simulink model "SensorModel"  (R2026a)
settings: Solver=FixedStepAuto  StartTime=0  StopTime=1000  FixedStep=0.1
model workspace (MAT data in the model file):
  SL_ROS_VariableLengthArrays_MaxSizes.CommonInfo.ArrayTruncateAction = 'EmitWarning'
  SL_ROS_VariableLengthArrays_MaxSizes.MsgTypeMap = containers.Map
  SL_ROS_VariableLengthArrays_MaxSizes.MsgTypeMap.serialization.keys = {'sensor_msgs/PointCloud2'}
  SL_ROS_VariableLengthArrays_MaxSizes.MsgTypeMap.serialization.values{1}(1).PropertyName = 'data'
  SL_ROS_VariableLengthArrays_MaxSizes.MsgTypeMap.serialization.values{1}(1).DataType = 'uint8'
  SL_ROS_VariableLengthArrays_MaxSizes.MsgTypeMap.serialization.values{1}(1).MaxLength = 4915200
  SL_ROS_VariableLengthArrays_MaxSizes.MsgTypeMap.serialization.values{1}(2).PropertyName = 'fields'
  SL_ROS_VariableLengthArrays_MaxSizes.MsgTypeMap.serialization.values{1}(2).DataType = 'sensor_msgs/PointField'
  SL_ROS_VariableLengthArrays_MaxSizes.MsgTypeMap.serialization.values{1}(2).MaxLength = 16
  SL_ROS_VariableLengthArrays_MaxSizes.MsgTypeMap.serialization.uniformity = 0
  SL_ROS_VariableLengthArrays_MaxSizes.MsgTypeMap.serialization.keyType = 'char'
  SL_ROS_VariableLengthArrays_MaxSizes.MsgTypeMap.serialization.valueType = 'any'
undefined symbols (not defined in the file): Defined, Ego, Lane, matlabshared, Sim3dSensor, simStepSize, User
libraries: roadrunnerscenario x6, drivingscenarioandsensors x2, ros2lib x2, sensoridealgroundtruthlib x1, sim3dcameralib x1, sim3dlib x1, sim3dautolib x1
settings Model: Creator=The MathWorks, Inc.  LastModifiedBy=akshran
settings DataIOCC: MaxDataPoints=100  SaveFormat=StructureWithTime  DatasetSignalFormat=timetable
settings DebuggingCC: SubsystemReferenceDiagnosticForUnitTest=warning
settings RTWCC: SystemTargetFile=ert.tlc  HardwareBoard=Robot Operating System 2 (ROS 2)  TLCOptions="-aInlineSetEventsForThisBaseRateFcn=TLC_FALSE -aSuppressMultiTaskScheduler=TLC_FALSE  -aRateBasedStepFcn=0"  Toolchain=Colcon Tools  TargetLang=C++  Description=Embedded Coder
settings ERTTargetCC: ExtModeTransport=2.0  ExtModeAutomaticAllocSize=off  RootIOFormat=Structure reference  CodeInterfacePackaging=C++ class

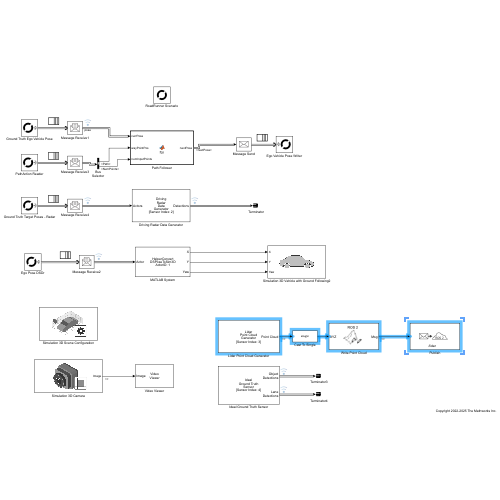
[thumbnail: Simulink's stored preview of the top-level diagram]
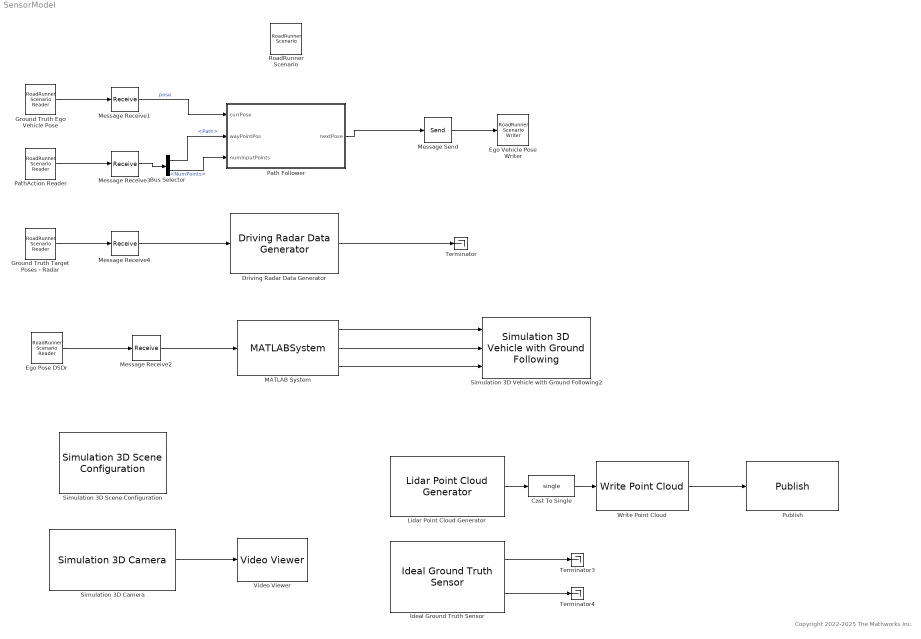
== system SensorModel ==
  note: Copyright 2022-2025 The Mathworks Inc.
  Bus Selector : BusSelector  OutputSignals=PathTarget.Path,PathTarget.NumPoints
  Cast To Single : DataTypeConversion  OutDataTypeStr=single  SaturateOnIntegerOverflow=off  RndMeth=Floor
  Driving Radar Data Generator : drivingscenarioandsensors/Driving Radar Data Generator  SensorIndex=2  UpdateRate=1/simStepSize  MountingLocation=[1.8, 0, 0.2 ]  MountingAngles=[0 0 0]  HasElevation=off  HasRangeRate=on  HasNoise=on  HasFalseAlarms=on  HasOcclusion=on  MaxNumReportsSource=Property  MaxNumReports=50  TargetReportFormat=Detections  DetectionCoordinates=Body  TrackCoordinates=Body  BusNameSource=Auto  BusName=BusDrivingRadarDataGenerator  SimulateUsing=Interpreted execution  AzimuthResolution=1  ElevationResolution=5  RangeResolution=2.5  RangeRateResolution=0.5  AzimuthBiasFraction=0.1  ElevationBiasFraction=0.1  RangeBiasFraction=0.05  RangeRateBiasFraction=0.05  FieldOfView=[ 80, 5 ]  RangeLimits=[ 0, 150 ]  RangeRateLimits=[ -100, 100 ]  DetectionProbability=0.9  FalseAlarmRate=1e-06  ReferenceRange=100  ReferenceRCS=0  CenterFrequency=77e9  FilterInitializationFcn=initcvekf  ConfirmationThreshold=[2 3]  DeletionThreshold=[5 5]  InitialSeedSource=Repeatable  InitialSeed=0  UsedSeed=matlabshared.tracking.internal.SimulinkUtilities.seedManager(gcb)  ProfilesSource=From Scenario Reader block  ProfilesParameters=driving.internal.ActorProfilesRadarParameters  ProfilesExpression=struct('ClassID',0,'Length',4.7,'Width',1.8,'Height',1.4,'OriginOffset',[-1.35 0 0],'RCSPattern',[10 10;10 10],'RCSAzimuthAngles',[-180 180],'RCSElevationAngles',[-90 90])
  Ego Pose DSDr : roadrunnerscenario/RoadRunner Scenario Reader  TopicCategory=Actor  ActorCategory=All Types  ActionType=Path Following  EventType=User-Defined  TopicType=Actor Pose (Driving Scenario compatible)  VehicleType=Vehicle Specifications  TrafficSignalType=Traffic Signal Specifications  TrafficSignalControllerType=Traffic Signal Controller Specifications  UserDefinedAction=Action1  UserDefinedEvent=Event1  Filter=Self  AdditionalRelationship=None  SensorTopic=Target Poses  LaneBoundaryOutputTopic=Ego-Lane  SensorID=1  SampleTime=0.1
  Ego Vehicle Pose Writer : roadrunnerscenario/RoadRunner Scenario Writer  TopicCategory=Actor  ActorCategory=All Types  EventType=Action Complete  UserDefinedEvent=Event1  VehicleType=Vehicle Pose  TopicType=Actor Pose
  Ground Truth Ego Vehicle Pose : roadrunnerscenario/RoadRunner Scenario Reader  TopicCategory=Actor  ActorCategory=All Types  ActionType=Path Following  EventType=User-Defined  TopicType=Actor Pose  VehicleType=Vehicle Pose  TrafficSignalType=Traffic Signal Specifications  TrafficSignalControllerType=Traffic Signal Controller Specifications  UserDefinedAction=Action1  UserDefinedEvent=Event1  Filter=Self  AdditionalRelationship=None  SensorTopic=Target Poses  LaneBoundaryOutputTopic=Ego-Lane  SensorID=1  SampleTime=0.1
  Ground Truth Target Poses - Radar : roadrunnerscenario/RoadRunner Scenario Reader  TopicCategory=Sensor  ActorCategory=All Types  ActionType=Path Following  EventType=User-Defined  TopicType=Actor Specifications  VehicleType=Vehicle Specifications  TrafficSignalType=Traffic Signal Specifications  TrafficSignalControllerType=Traffic Signal Controller Specifications  UserDefinedAction=Action1  UserDefinedEvent=Event1  Filter=Self  AdditionalRelationship=None  SensorTopic=Target Poses  LaneBoundaryOutputTopic=Ego-Lane  SensorID=2  SampleTime=0.1
  Ideal Ground Truth Sensor : sensoridealgroundtruthlib/Ideal Ground Truth Sensor  SensorIndex=4  DetectorOutput=Objects and Lanes  UpdateInterval=simStepSize  SensorLocation=[ 1.9, 0, 0.2 ]  Yaw=0  Pitch=0  Roll=0  FieldOfView=[ 120, 30 ]  MaxRange=50  DetectionCoordinates=Host Coordinates  PointOnTargetReported=Origin Point  TargetOutputFormat=Object Detections  MaxNumObjectDetections=300  LaneBoundariesReported=All Lanes  MaxNumLaneDetections=300  BusNameSource=Auto  BusName=BusSSFGroundTruthObjects  BusName2Source=Auto  BusName2=BusSSFGroundTruthLaneBoundaries  SimulateUsing=Interpreted execution
  Lidar Point Cloud Generator : drivingscenarioandsensors/Lidar Point Cloud Generator  SensorIndex=3  UpdateInterval=simStepSize  SensorLocation=[1.5 0]  Height=1.6  Yaw=0  Pitch=0  Roll=0  DetectionCoordinates=Ego Cartesian  HasEgoVehicle=on  EgoVehicleActorID=1  HasRoadsInputPort=on  ActorProfilesSource=From Scenario Reader block  ActorProfilesVariableName=actor_profiles  MaxRange=120  RangeAccuracy=0.002  AzimuthResolution=0.16  ElevationResolution=1.25  AzimuthLimits=[ -180, 180 ]  ElevationLimits=[ -20, 20 ]  HasNoise=on
  MATLAB System : MATLABSystem  System=HelperConvertDSPoseToSim3D  ActorProfiles=struct( 'ActorID', 1, 'ClassID', 1, 'Length', 4.7, 'Width', 1.8, 'Height', 1.4, 'OriginOffset', [ 0, 0, 0 ], 'FrontOverhang', 0, 'RearOverhang', 0, 'Wheelbase', 0, 'Color', [ 0, 0, 0 ] )  ActorIDToConvert=1  SimulateUsing=Code generation
      mask Type: HelperConvertDSPoseToSim3D
  Message Receive{1..4} (4 alike) : Receive  InputPortMessageModes=m  UseInternalQueue=off  SampleTime=simStepSize
  Message Send : Send  OutputPortMessageModes=m
  Path Follower : MATLAB Function  TreatAsAtomicUnit=on
  PathAction Reader : roadrunnerscenario/RoadRunner Scenario Reader  TopicCategory=Action  ActorCategory=All Types  ActionType=Path Following  EventType=User-Defined  TopicType=Actor Specifications  VehicleType=Vehicle Specifications  TrafficSignalType=Traffic Signal Specifications  TrafficSignalControllerType=Traffic Signal Controller Specifications  UserDefinedAction=Action1  UserDefinedEvent=Event1  Filter=Self  AdditionalRelationship=None  SensorTopic=Target Poses  LaneBoundaryOutputTopic=Ego-Lane  SensorID=1  SampleTime=0.1
  Publish : ros2lib/Publish  topicSource=Specify your own  topic=/lidar  messageType=sensor_msgs/PointCloud2  QOSHistory=Keep last  QOSDepth=10  QOSReliability=Reliable  QOSDurability=Volatile  QOSDeadline=Inf  QOSLifespan=Inf  QOSLiveliness=Automatic  QOSLeaseDuration=Inf  QOSAvoidROSNamespaceConventions=off
  RoadRunner Scenario : roadrunnerscenario/RoadRunner Scenario  ScenarioFileName=C:\Users\akshran\OneDrive - MathWorks\Documents\EIC_RR1\EIC_FW\Scenarios\EIC  ActorIDLinkedToModel=1  SampleTime=0.1  OpenRoadRunnerAtSimulationStart=on  EnableSimulationLoggingInRoadRunner=on  UserDefinedActions={}  UserDefinedEvents={}  PathPoints=500
  Simulation 3D Camera : sim3dcameralib/Simulation 3D Camera  Priority=1  sensorTag=Sim3dSensor�  sensorId=1  sensorName=Sim3dSensor�  vehTagList={'Custom ...';'Scene Origin';'SimulinkVehicle1'}  vehTag=SimulinkVehicle1  CoordinateSystem=ISO8855  mountLoc=Roof center  offsetFlag=off  tmountOffset=[0, 0, 0]  extTmount=off  rmountOffset=[0, 0, 0]  extRmount=off  FocalLength=[1109, 1109]  OpticalCenter=[640, 360]  ImageSize=[720, 1280]  RadialDistortion=[0, 0]  TangentialDistortion=[0, 0]  SensorSkew=0  VisualizeFieldOfView=off  FieldOfViewRange=61  DepthOutportEnabled=off  SemanticOutportEnabled=off  TransformOutportEnabled=off  SampleTime=-1  mountPoint=[-0.45 0 1.68]  mountOrientation=[0 0 0]  aMode=3  ID=1
      settings: LibrarySourceBlock=drivingsim3d/Simulation 3D Camera
  Simulation 3D Scene Configuration : sim3dlib/Simulation 3D Scene Configuration  Priority=0  ProjectFormat=RoadRunner  SceneDesc=Straight road  ProjectName=C:\Program Files\MATLAB\R2026a\toolbox\shared\sim3d_projects\automotive_project_windows\UE\WindowsNoEditor\VehicleSimulation.exe  ScenePath=/Game/Maps/HwStrght  RoadRunnerProjectPath=C:\Users\akshran\OneDrive - MathWorks\Documents\EIC_RR1\EIC_FW\Exports\EIC.fbx  EnableOpenDRIVE=off  vehTagList={'Custom';'Scene Origin';'SimulinkVehicle1'}  vehTag=SimulinkVehicle1  AttachedCameraRelativeTranslation=[0 0 0]  FreeCameraDefaultInitialTranslation=[-6, 0, 2]  AttachedCameraRelativeRotation=[0, -15, 0]  FreeCameraDefaultInitialRotation=[0, -15, 0]  ViewpointName=Custom  FreeCameraInitialTranslation=[0, 0, 0]  FreeCameraInitialRotation=[0, 0, 0]  OpVisEn=off  Ts=0.1  EnableWindow=on  EnableRemoteAccess=off  SimulationMode=CoSimulation  SimulateUsing=Interpreted execution  EnableAnimationRecording=off  OverrideDefaultRecording=off  AnimationRecordingFileName=sim3dAnimation.mat  AnimationRecordingInterval=[0 inf]  EnableWeather=off  SunAzimuth=90  SunAltitude=40.0  EnableGeospatialSun=off  Latitude=0  Longitude=0  Date=2023-01-01  Time=10:30:00  GeoTimeZone=-5.0  SunDaylightSaving=off  wind=1  clouds=10  EnableVolumetricClouds=off  CloudCoverage=0  CloudAltitude=6  fog=0  rain=0  RaindropsEffect=off  SnowDensity=0  EnableGeospatial=off  TilesetSource=Earth terrain  UseTrueOrigin=off  OriginHeight=200  OriginLatitude=40.744652  OriginLongitude=-73.988864  MapStyle=Aerial  AdditionalAssetIDs=[]  UseAdvancedSunSky=off  SolarTime=11  TimeZone=-5  Day=21  Month=9  Year=2022  UseDaylightSavingTime=on  DSTStartDay=10  DSTStartMonth=3  DSTEndDay=3  DSTEndMonth=11  DSTSwitchHour=2  sensorTag=MainCamera1  sensorId=1  sensorName=MainCamera1  mountLoc=Origin  offsetFlag=off  tmountOffset=[0, 0, 0]  rmountOffset=[0, 0, 0]  HorizontalResolution=1280  VerticalResolution=720  HorizontalFOV=60  mountPoint=[0 0 0]  mountOrientation=[0 0 0]  aMode=3  ID=1  GeoTrigger=Inactive  ViewNameList={'Custom'}  ViewTranslationList={'[0 0 0]'}  ViewRotationList={'[0 0 0]'}
      settings: LibrarySourceBlock=drivingsim3d/Simulation 3D Scene Configuration
  Simulation 3D Vehicle with Ground Following2 : sim3dautolib/Simulation 3D Vehicle with Ground Following  Priority=-1  PassVehMesh=Sedan  MeshPath=/MathWorksAutomotiveContent/Vehicles/Muscle/Meshes/SK_MuscleCar.SK_MuscleCar  TrackWidth=1.9  WheelBase=3  WheelRadius=0.35  VehColor=Silver  CoordinateSystem=ISO8855  InitialPos=[-7.539,-70.4747,0]  InitialRot=[0, 0, 0]  ActorName=SimulinkVehicle1  SampleTime=-1  ActorType=SimulinkVehicle  ID=1  aMode=3  ActorTag=SimulinkVehicle1  CoordinateScheme=0  VehLightsControl=off  HeadlightColor=[ 1, 1, 1 ]  HighBeamIntensity=100000  LowBeamIntensity=60000  HighBeamConeAngle=70  LowBeamConeAngle=70  LeftHeadlightOrientation=[ 0, 0 ]  RightHeadlightOrientation=[ 0, 0 ]  BrakelightIntensity=500  ReverselightIntensity=500  SignallightIntensity=500  SignallightPeriod=1  SignalPulseWidth=50  TransformOutportEnabled=off
      settings: LibrarySourceBlock=drivingsim3d/Simulation 3D Vehicle with Ground Following
  Terminator : Terminator
  Terminator3 : Terminator
  Terminator4 : Terminator
  Video Viewer : VideoViewer  FigPos=[431 551 418 304]
  Write Point Cloud : ros2lib/Write Point Cloud  messageType=sensor_msgs/PointCloud2  Encoding=none  HasRGB=false  HasAlpha=false  HasIntensityCheck=off  HasIntensity=false  FieldNamesStruct=struct('x', 'single', 'y', 'single', 'z', 'single')
  wires:
  Ground Truth Ego Vehicle Pose/1 -> Message Receive1/1
  Path Follower/1(nextPose) -> Message Send/1
  Message Receive1/1 -> Path Follower/1(currPose)  "pose"
  PathAction Reader/1 -> Message Receive3/1
  Message Receive3/1 -> Bus Selector/1
  Message Send/1 -> Ego Vehicle Pose Writer/1
  Bus Selector/1 -> Path Follower/2(wayPointPos)  "<Path>"
  Driving Radar Data Generator/1 -> Terminator/1
  Ground Truth Target Poses - Radar/1 -> Message Receive4/1
  Message Receive4/1 -> Driving Radar Data Generator/1
  Lidar Point Cloud Generator/1 -> Cast To Single/1
  Ideal Ground Truth Sensor/1 -> Terminator3/1
  Ideal Ground Truth Sensor/2 -> Terminator4/1
  Bus Selector/2 -> Path Follower/3(numInputPoints)  "<NumPoints>"
  Simulation 3D Camera/1 -> Video Viewer/1
  Write Point Cloud/1 -> Publish/1
  Cast To Single/1 -> Write Point Cloud/1
  Message Receive2/1 -> MATLAB System/1
  Ego Pose DSDr/1 -> Message Receive2/1
  MATLAB System/1 -> Simulation 3D Vehicle with Ground Following2/1
  MATLAB System/2 -> Simulation 3D Vehicle with Ground Following2/2
  MATLAB System/3 -> Simulation 3D Vehicle with Ground Following2/3

== matlab function SensorModel/Path Follower ==
  data: currPose input; wayPointPos input; numInputPoints input; nextPose output Bus: BusActorRuntime; simStepSize parameter
function nextPose    = fcn(currPose, wayPointPos, numInputPoints, simStepSize)

% Set constant ego vehicle speed
egoSpeed  = 18;

% Declare persistent variables for simulation and retain only non zero
% elements in the array of waypoints 
persistent wayPointIdx wayPointPosInterp headingAnglesInterp numWayPoints
wayPointPos = wayPointPos(1:numInputPoints,:);

% Extract poses for the entire path before simulation begins
if isempty(wayPointIdx)
    
    wayPointIdx = 2;

    % Pre-allocate arrays
    wayPointPosInterp = [];
    headingAnglesInterp = [];

    % Get heading angle
    startHeadingAngle = atan2d(-currPose.Pose(1,2),currPose.Pose(1,1));
  
     % Calculate distance from the each waypoint to the next waypoint
    delXY = diff(wayPointPos(:,[1 2]));
    absDistToNextPoints = sqrt(delXY(:,1).^2 + delXY(:,2).^2);

    % Calculate time of arrival at the next wayPoint based on the
    % set constant speed. Alternatively, you can set the timing profile
    % in RoadRunner for waypoints and use those here 
    trueTimes = [0;cumsum(absDistToNextPoints/egoSpeed)];

    % Calculate the heading angle to proceed towards each waypoint
    headingAngles = [startHeadingAngle;atan2d(delXY(:,2),delXY(:,1))-90];

    % Calculate time of arrival at all the wayPoints based on the
    % simulation step size and use it for final interpolation.
    globalTimeVec = 0:simStepSize:trueTimes(end);

    % Interpolate X and Y positions between all waypoints
    % along the entire time vector and store them
    interpPosPointsX = interp1(trueTimes,wayPointPos(:,1),globalTimeVec)';
    interpPosPointsY = interp1(trueTimes,wayPointPos(:,2),globalTimeVec)';
    wayPointPosInterp = [interpPosPointsX interpPosPointsY];

    % Interpolate heading angles between the all waypoints
    % along the entire time vector and store them
    headingAnglesInterp = interp1(trueTimes,headingAngles,globalTimeVec');

    % Get the new total number of waypoints after interpolation
    numWayPoints = length(wayPointPosInterp);
end

% At each time step of the simulation, send the next waypoint position from the
% interpolated waypoint array until ego vehicle arrives at the last waypoint
nextPose = currPose;
nextPose.Pose(1,4) = wayPointPosInterp(wayPointIdx,1);
nextPose.Pose(2,4) = wayPointPosInterp(wayPointIdx,2);

% Convert the heading angle (yaw) to a rotation matrix
nextPose.Pose(1:3,1:3) = [cosd(headingAnglesInterp(wayPointIdx)) -sind(headingAnglesInterp(wayPointIdx)) 0;...
                          sind(headingAnglesInterp(wayPointIdx)) cosd(headingAnglesInterp(wayPointIdx)) 0;...
                          0 0 1];


if(wayPointIdx<numWayPoints)
    wayPointIdx = wayPointIdx + 1;
end

end
